simulink model "Equal_1"  (R2018a)
settings: Solver=VariableStepAuto  StartTime=0.0  StopTime=10.0  RelTol=1e-3
settings Model: Creator=midog  LastModifiedBy=midog

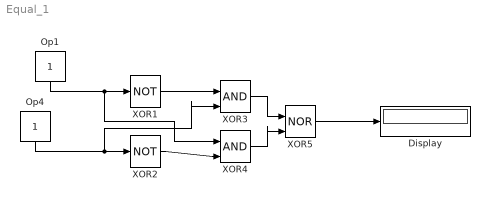
== system Equal_1 ==
  Display : Display
  Op1 : Constant
  Op4 : Constant
  XOR1 : Logic  Operator=NOT  IconShape=distinctive  AllPortsSameDT=off  OutDataTypeStr=boolean
  XOR2 : Logic  Operator=NOT  IconShape=distinctive  AllPortsSameDT=off  OutDataTypeStr=boolean
  XOR3 : Logic  IconShape=distinctive  AllPortsSameDT=off  OutDataTypeStr=boolean
  XOR4 : Logic  IconShape=distinctive  AllPortsSameDT=off  OutDataTypeStr=boolean
  XOR5 : Logic  Operator=NOR  IconShape=distinctive  AllPortsSameDT=off  OutDataTypeStr=boolean
  wires:
  Op4/1 -> XOR3/2, XOR2/1
  Op1/1 -> XOR4/1, XOR1/1
  XOR1/1 -> XOR3/1
  XOR3/1 -> XOR5/1
  XOR4/1 -> XOR5/2
  XOR2/1 -> XOR4/2
  XOR5/1 -> Display/1
